simulink model "xuanjia"  (R2016b)
settings: Solver=VariableStepAuto  StartTime=0.0  StopTime=10.0  RelTol=1e-3
settings Model: Creator=Administrator  LastModifiedBy=yehoo
settings DataIOCC: LimitDataPoints=on  SaveOutput=off  SaveTime=off
settings OptimizationCC: BlockReduction=off  BooleanDataType=off  LifeSpan=inf
settings DebuggingCC: SaveWithParameterizedLinksMsg=none  UnderspecifiedInitializationDetection=Classic  MergeDetectMultiDrivingBlocksExec=none  SignalResolutionControl=TryResolveAllWithWarning  AllowSymbolicDim=off  SFUnexpectedBacktrackingDiag=warning  SFNoUnconditionalDefaultTransitionDiag=warning  SFExecutionAtInitializationDiag=none
settings HardwareCC: TargetUnknown=on
settings GRTTargetCC: TargetLangStandard=C89/C90 (ANSI)  GeneratePreprocessorConditionals=Disable all
settings ConfigComp: CovMetricSettings=dw  CovHtmlReporting=on  CovSaveCumulativeToWorkspaceVar=on  CovSaveSingleToWorkspaceVar=on  CovExternalEMLEnable=off

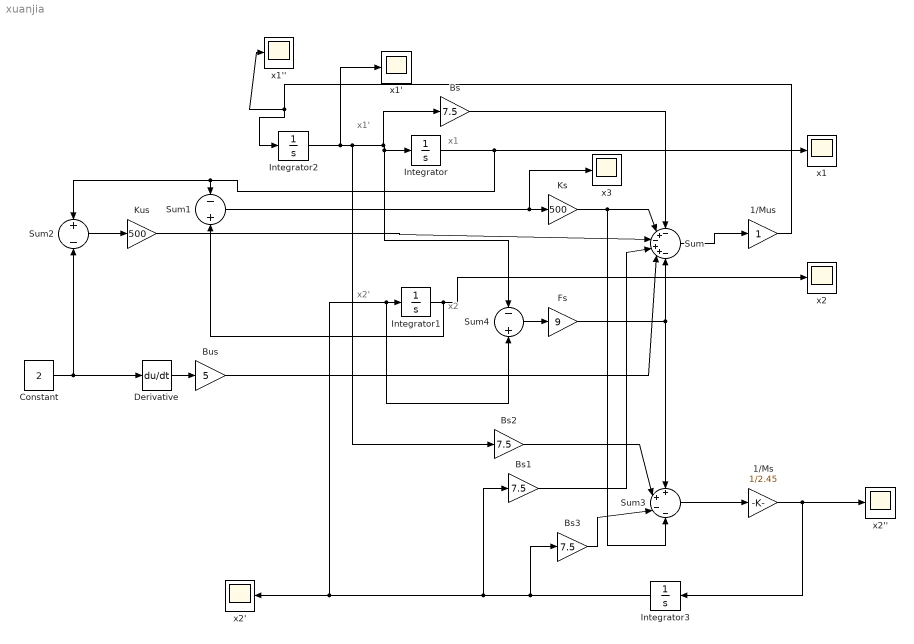
== system xuanjia ==
  note: x1
  note: x1'
  note: x2
  note: x2'
  1/Ms : Gain  Gain=1/2.45
  1/Mus : Gain
  Bs{,1..3} (4 alike) : Gain  Gain=7.5
  Bus : Gain  Gain=5
  Constant : Constant  Value=2
  Derivative : Derivative
  Fs : Gain  Gain=9
  Integrator{,1..3} (4 alike) : Integrator
  Ks : Gain  Gain=500
  Kus : Gain  Gain=500
  Sum : Sum  Inputs=-+-++-
  Sum1 : Sum  Inputs=-+
  Sum2 : Sum  Inputs=+-
  Sum3 : Sum  Inputs=++--
  Sum4 : Sum  Inputs=-+
  x1 : Scope
  x1' : Scope
  x1'' : Scope
  x2 : Scope
  x2' : Scope
  x2'' : Scope
  x3 : Scope
  wires:
  Integrator2/1 -> Sum4/1, Integrator/1, Bs/1, Bs2/1, x1'/1
  Bs/1 -> Sum/1
  Integrator3/1 -> x2'/1, Sum4/2, Integrator1/1, Bs1/1, Bs3/1
  1/Ms/1 -> Integrator3/1, x2''/1
  Integrator1/1 -> x2/1, Sum1/2
  Ks/1 -> Sum/2, Sum3/4
  Bs1/1 -> Sum/4
  Bus/1 -> Sum/5
  Constant/1 -> Derivative/1, Sum2/2
  Integrator/1 -> Sum2/1, Sum1/1, x1/1
  Sum2/1 -> Kus/1
  Kus/1 -> Sum/3
  Bs2/1 -> Sum3/2
  Bs3/1 -> Sum3/3
  Derivative/1 -> Bus/1
  Sum3/1 -> 1/Ms/1
  Sum/1 -> 1/Mus/1
  1/Mus/1 -> x1''/1, Integrator2/1
  Sum4/1 -> Fs/1
  Fs/1 -> Sum3/1, Sum/6
  Sum1/1 -> x3/1, Ks/1
